simulink model "SimulinkModel"  (R2022a)
settings: Solver=VariableStepAuto  StartTime=0.0  StopTime=500  RelTol=1e-3
settings Model: Creator=Kulith  LastModifiedBy=Kulith

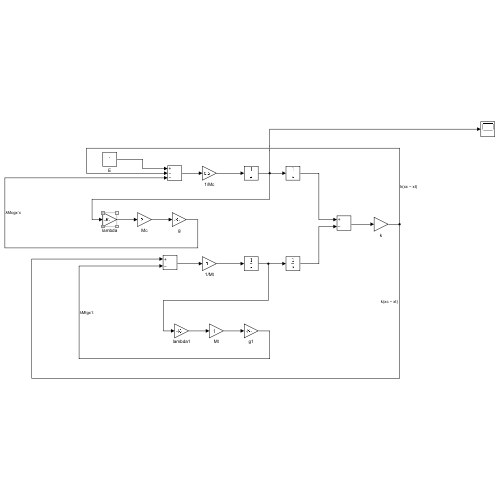
[thumbnail: Simulink's stored preview of the top-level diagram]
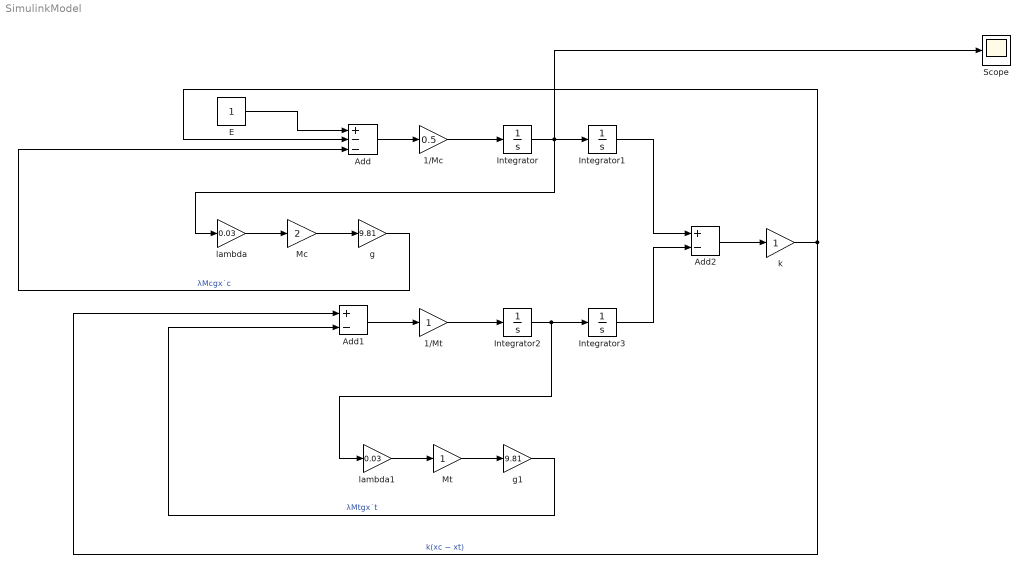
== system SimulinkModel ==
  1/Mc : Gain  Gain=0.5
  1/Mt : Gain
  Add : Sum  Inputs=+--
  Add1 : Sum  Inputs=+-
  Add2 : Sum  Inputs=+-
  E : Constant
  Integrator{,1..3} (4 alike) : Integrator
  Mc : Gain  Gain=2
  Mt : Gain
  Scope : Scope
  g : Gain  Gain=9.81
  g1 : Gain  Gain=9.81
  k : Gain
  lambda : Gain  Gain=0.03
  lambda1 : Gain  Gain=0.03
  wires:
  Add2/1 -> k/1
  Integrator1/1 -> Add2/1
  g1/1 -> Add1/2  "λMtgx˙t"
  Mt/1 -> g1/1
  Mc/1 -> g/1
  lambda/1 -> Mc/1
  Integrator2/1 -> lambda1/1, Integrator3/1
  1/Mc/1 -> Integrator/1
  lambda1/1 -> Mt/1
  Add/1 -> 1/Mc/1
  Integrator3/1 -> Add2/2
  g/1 -> Add/3  "λMcgx˙c"
  Integrator/1 -> Scope/1, lambda/1, Integrator1/1
  k/1 -> Add1/1, Add/2  "k(xc − xt)"
  Add1/1 -> 1/Mt/1
  1/Mt/1 -> Integrator2/1
  E/1 -> Add/1
